simulink model "ballbeam_sim"  (Simulink 8.3)
settings: Solver=ode45  StartTime=0.0  StopTime=100  RelTol=1e-3
undefined symbols (not defined in the file or in its folder): AP, drawBallBeam
settings Model: Creator=beard  LastModifiedBy=jhl48
settings OptimizationCC: ExpressionDepthLimit=2147483647  InitFltsAndDblsToZero=on
settings DebuggingCC: FcnCallInpInsideContextMsg=UseLocalSettings

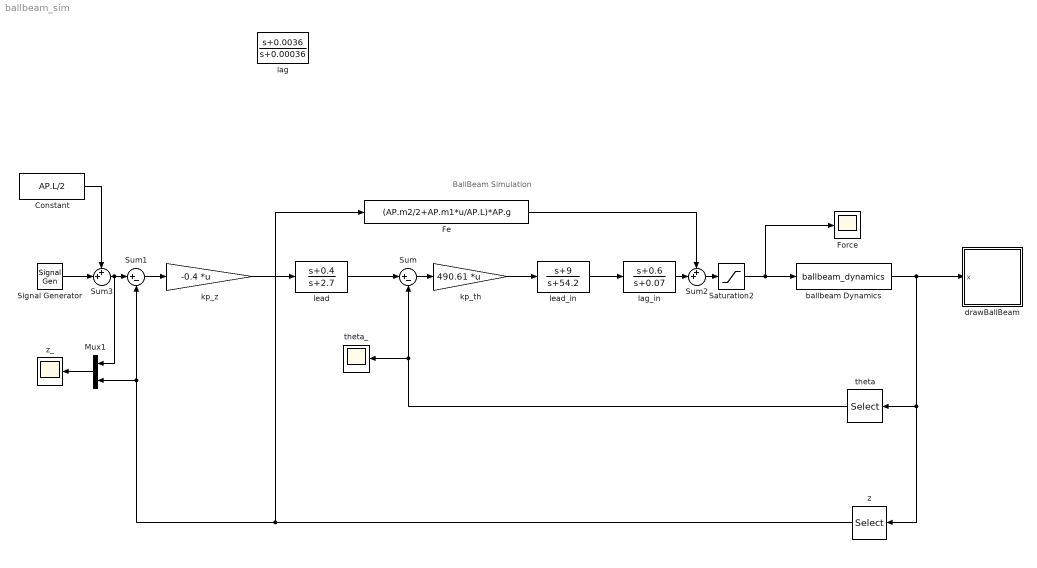
== system ballbeam_sim ==
  note: BallBeam Simulation
  Constant : Constant  Value=AP.L/2
  Fe : Fcn  Expr=(AP.m2/2+AP.m1*u/AP.L)*AP.g
  Force : Scope
      settings: TimeRange=100  YMin=7  YMax=15
  Mux1 : Mux  Inputs=2
  Saturation2 : Saturate  UpperLimit=50  LowerLimit=-50
  Signal Generator : SignalGenerator  WaveForm=square  Amplitude=.15  Frequency=.1  Units=rad/sec
  Sum : Sum  Inputs=|+-
  Sum1 : Sum  Inputs=|+-
  Sum2 : Sum  Inputs=++|
  Sum3 : Sum  Inputs=++|
  ballbeam Dynamics : S-Function  FunctionName=ballbeam_dynamics  Parameters=AP  EnableBusSupport=off
  drawBallBeam : Subsystem
      mask init:
      | % drawing parameters
      | L = .5;
      | R = L/10;
      mask Display: image(imread('tv.jpg'))
  kp_th : Gain  Gain=490.61  Multiplication=Matrix(K*u)
  kp_z : Gain  Gain=-0.4  Multiplication=Matrix(K*u)
  lag : TransferFcn  Numerator=[1 0.0036]  Denominator=[1 0.00036]
  lag_in : TransferFcn  Numerator=[1 0.6]  Denominator=[1 0.07]
  lead : TransferFcn  Numerator=[1 0.4]  Denominator=[1 2.7]
  lead_in : TransferFcn  Numerator=[1 9]  Denominator=[1 54.2]
  theta : Selector  InputPortWidth=4  Indices=[1]
  theta_ : Scope
      settings: TimeRange=100  YMin=-0.02  YMax=0.0225
  z : Selector  InputPortWidth=4  Indices=[2]
  z_ : Scope
      settings: TimeRange=100  YMin=2.77556e-17  YMax=0.5  SaveName=ScopeData2
  wires:
  ballbeam Dynamics/1 -> drawBallBeam/1(x), theta/1, z/1
  Sum2/1 -> Saturation2/1
  Sum/1 -> kp_th/1
  theta/1 -> Sum/2, theta_/1
  z/1 -> Fe/1, Sum1/2, Mux1/2
  Mux1/1 -> z_/1
  Sum1/1 -> kp_z/1
  Saturation2/1 -> ballbeam Dynamics/1, Force/1
  kp_z/1 -> lead/1
  kp_th/1 -> lead_in/1
  lead_in/1 -> lag_in/1
  lag_in/1 -> Sum2/2
  Fe/1 -> Sum2/1
  lead/1 -> Sum/1
  Constant/1 -> Sum3/1
  Signal Generator/1 -> Sum3/2
  Sum3/1 -> Mux1/1, Sum1/1

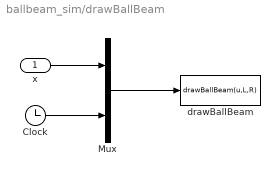
== system ballbeam_sim/drawBallBeam ==
  x : Inport
  Clock : Clock
  Mux : Mux  Inputs=2
  drawBallBeam : MATLABFcn  MATLABFcn=drawBallBeam(u,L,R)  OutputDimensions=0  SampleTime=0.01
  wires:
  Mux/1 -> drawBallBeam/1
  x/1 -> Mux/1
  Clock/1 -> Mux/2
